simulink model "flythedrone"  (R2019b)
settings: Solver=FixedStepAuto  StartTime=0.0  StopTime=100  RelTol=1e-3
InitFcn:
  | load('BusDefinitions.mat')
values from neighbouring files (symbols this model uses):
  Kaileron = Kaileron(2:4)    [HW7_v2_matlab.m]
  Kelevator = Kelevator(2:4)    [HW7_v2_matlab.m]
  Krudder = Krudder(2)    [HW7_v2_matlab.m]
  Kthrust = lqr(Athrust, Bthrust, Qthrust, Rthrust)    [HW7_v2_matlab.m]
  M_motor = [1, 1, 1, -1;             1, 1, -1, 1;             1, -1, -1, -1;             1, -1, 1, 1 ]    [HW7_v2_matlab.m]
undefined symbols (not defined in the file or in its folder): A_s_double, A_s_single, B_s_double, B_s_single, C_double, C_single, codertarget, D_double, D_single, DiscIntNeverNeededParam, Discrete, omega_c, q_single, r_single, Time, Ts
libraries: ctrlSharedLib x5
settings Model: ExtModeTrigDuration=80  Creator=Sankalp Bhan  LastModifiedBy=cwhipp
settings OptimizationCC: PassReuseOutputArgsThreshold=0  MaxStackSize=64
settings DebuggingCC: ParameterTunabilityLossMsg=error  ArithmeticOperatorsInVariantConditions=warning
settings HardwareCC: ProdBitPerPointer=32  ProdBitPerSizeT=32  ProdBitPerPtrDiffT=32  ProdLargestAtomicInteger=Long  ProdWordSize=32  ProdHWDeviceType=ARM Compatible->ARM 9  UseEmbeddedCoderFeatures=off
settings SFSimCC: SimUseLocalCustomCode=off  MATLABDynamicMemAlloc=off
settings RTWCC: SystemTargetFile=ert.tlc  HardwareBoard=PARROT Mambo  TLCOptions="-aInlineSetEventsForThisBaseRateFcn=TLC_FALSE -aSuppressMultiTaskScheduler=TLC_FALSE   -aRateBasedStepFcn=1"  TemplateMakefile=ert_default_tmf  GenerateReport=on  RTWUseLocalCustomCode=off  Toolchain=Sourcery G++ Lite GNU Toolchain for Drones  LaunchReport=on
settings CodeAppCC: ForceParamTrailComments=on  OperatorAnnotations=on  StateflowObjectComments=on
settings ERTTargetCC: ERTCustomFileBanners=off  MatFileLogging=on  SupportContinuousTime=on  SupportNonInlinedSFcns=on  RemoveResetFunc=off  ModelStepFunctionPrototypeControlCompliant=off

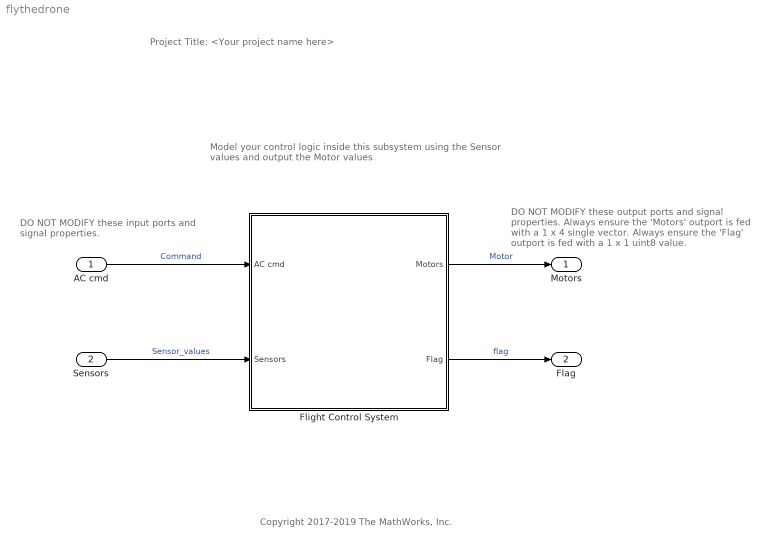
== system flythedrone ==
  note: Model your control logic inside this subsystem
      | using the Sensor values and output the
      | Motor values
  note: DO NOT MODIFY these output ports
      | and signal properties.
      |
      |
      |
      | Always ensure the 'Motors' outport
      | is fed with a 1 x 4 single vector.
      |
      |
      |
      |
      |
      | Always ensure the 'Flag' outport is
      | fed with a 1 x 1 uint8 value.
  note: DO NOT MODIFY these input
      | ports and signal properties.
  note: Copyright 2017-2019 The MathWorks, Inc.
  note: Project Title: <Your project name here>
  AC cmd : Inport  OutDataTypeStr=Bus: CommandBus  BusOutputAsStruct=on
  Sensors : Inport  Port=2  OutDataTypeStr=Bus: SensorsBus  BusOutputAsStruct=on
  Flight Control System : Subsystem  InitFcn=codertarget.parrot.internal.fcsSubsystemCallback(gcb);
  Motors : Outport  OutDataTypeStr=single  PortDimensions=[1 4]  VectorParamsAs1DForOutWhenUnconnected=off
  Flag : Outport  Port=2  OutDataTypeStr=uint8  PortDimensions=1  VectorParamsAs1DForOutWhenUnconnected=off
  wires:
  Flight Control System/1(Motors) -> Motors/1  "Motor"
  AC cmd/1 -> Flight Control System/1(AC cmd)  "Command"
  Sensors/1 -> Flight Control System/2(Sensors)  "Sensor_values"
  Flight Control System/2(Flag) -> Flag/1  "flag"

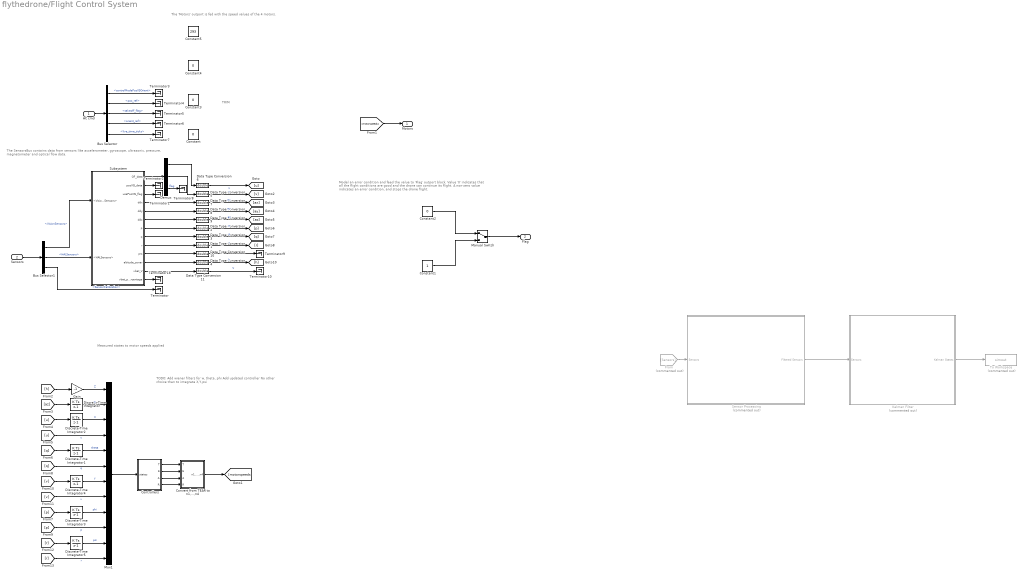
== system flythedrone/Flight Control System ==
  note: TODO:
      | Add wiener filters for w, theta, phi
      | Add updated controller
      |
      | No other choice than to integrate X,Y,psi
  note: Measured states to motor speeds applied
  note: TRIM
  note: The 'Motors' outport is fed with the speed values of the 4 motors.
  note: Model an error condition and feed the value to 'Flag' outport block.
      | Value '0' indicates that all the flight conditions are good and the drone
      | can continue its flight.
      | A non-zero value indicates an error condition, and stops the drone
      | flight.
  note: The SensorsBus contains data from sensors like
      | accelerometer, gyroscope, ultrasonic, pressure,
      | magnetometer and optical flow data.
  AC cmd : Inport
  Sensors : Inport  Port=2
  Bus Selector : BusSelector  OutputSignals=controlModePosVSOrient,pos_ref,takeoff_flag,orient_ref,live_time_ticks
  Bus Selector1 : BusSelector  OutputSignals=VisionSensors,HALSensors,SensorCalibration
  Constant : Constant  Value=0  SampleTime=Ts
  Constant1 : Constant  OutDataTypeStr=uint8
  Constant2 : Constant  Value=0  OutDataTypeStr=uint8
  Constant3 : Constant  Value=0  SampleTime=Ts
  Constant4 : Constant  Value=0  SampleTime=Ts
  Constant5 : Constant  Value=293  SampleTime=Ts
  Controllers : Subsystem
  Convert from TEAR to n1,...,n4 : Subsystem
  Data Type Conversion{1..11} (11 alike) : DataTypeConversion  OutDataTypeStr=double
  Demux : Demux  Outputs=3
  Discrete-Time Integrator{,1..5} (6 alike) : DiscreteIntegrator  SampleTime=-1  ICPrevOutput=DiscIntNeverNeededParam  ICPrevScaledInput=DiscIntNeverNeededParam
  From : From  Commented=on  GotoTag=Sensors
  Gain : Gain  Gain=-1
  Kalman Filter : Subsystem  Commented=on
  Manual Switch : ManualSwitch
  Mux1 : Mux  Inputs=12
  "Sensor Processing " : Subsystem  Commented=on
  Subsystem : Subsystem
  Terminator{,1..10,18} (12 alike) : Terminator
  To Workspace : ToWorkspace  Commented=on  VariableName=simout  SaveFormat=Structure With Time  SampleTime=-1
  Motors : Outport  VectorParamsAs1DForOutWhenUnconnected=off
  Flag : Outport  Port=2  VectorParamsAs1DForOutWhenUnconnected=off
  wires:
  AC cmd/1 -> Bus Selector/1
  Sensors/1 -> Bus Selector1/1
  Bus Selector/1 -> Terminator3/1  "<controlModePosVSOrient>"
  Bus Selector/2 -> Terminator4/1  "<pos_ref>"
  Bus Selector/3 -> Terminator5/1  "<takeoff_flag>"
  Bus Selector/4 -> Terminator6/1  "<orient_ref>"
  Bus Selector/5 -> Terminator7/1  "<live_time_ticks>"
  Manual Switch/1 -> Flag/1
  Constant2/1 -> Manual Switch/1
  Constant1/1 -> Manual Switch/2
  [motorspeeds] -> Motors/1
  Bus Selector1/1 -> Subsystem/1(<VisionSensors>)  "<VisionSensors>"
  Bus Selector1/2 -> Subsystem/2(<HALSensors>)  "<HALSensors>"
  Bus Selector1/3 -> Terminator/1  "<SensorCalibration>"
  Subsystem/1(OF_data) -> Demux/1
  Subsystem/4(ddx) -> Data Type Conversion7/1
  Subsystem/5(ddy) -> Data Type Conversion8/1
  Subsystem/6(ddz) -> Data Type Conversion9/1
  Subsystem/7(p) -> Data Type Conversion2/1
  Subsystem/9(r) -> Data Type Conversion1/1
  Subsystem/11(altitude_sonar) -> Data Type Conversion4/1
  Subsystem/12(vbat_V) -> Data Type Conversion11/1
  Subsystem/13(vbat_percentage) -> Terminator18/1
  Subsystem/8(q) -> Data Type Conversion3/1
  Subsystem/3(usePosVIS_flag) -> Terminator1/1
  Subsystem/2(posVIS_data) -> Terminator2/1
  Demux/1 -> Data Type Conversion6/1
  Demux/2 -> Data Type Conversion5/1
  Demux/3 -> Terminator8/1  "flag"
  Subsystem/10(prs) -> Data Type Conversion10/1
  Data Type Conversion1/1 -> [r]  "r"
  Data Type Conversion2/1 -> [p]  "p"
  Data Type Conversion3/1 -> [q]  "q"
  Data Type Conversion4/1 -> [h]  "h"
  Data Type Conversion5/1 -> [v]  "v"
  Data Type Conversion6/1 -> [u]  "u"
  Data Type Conversion7/1 -> [ax]  "ax"
  Data Type Conversion8/1 -> [ay]  "ay"
  Data Type Conversion9/1 -> [az]  "az"
  Data Type Conversion10/1 -> Terminator9/1
  Data Type Conversion11/1 -> Terminator10/1  "V"
  From/1 -> "Sensor Processing "/1(Sensors)
  "Sensor Processing "/1(Filtered Sensors) -> Kalman Filter/1(Sensors)
  Kalman Filter/1(Kalman States) -> To Workspace/1
  Mux1/1 -> Controllers/1(states)
  Controllers/3(A) -> Convert from TEAR to n1,...,n4/3(A)
  Controllers/4(R) -> Convert from TEAR to n1,...,n4/4(R)
  Controllers/1(T) -> Convert from TEAR to n1,...,n4/1(T)
  Controllers/2(E) -> Convert from TEAR to n1,...,n4/2(E)
  Convert from TEAR to n1,...,n4/1(n1,...,n4) -> [motorspeeds]
  [h] -> Gain/1
  Gain/1 -> Mux1/1  "Z"
  [az] -> Discrete-Time Integrator/1
  Discrete-Time Integrator/1 -> Mux1/2  "w"
  [u] -> Mux1/4  "u"
  Discrete-Time Integrator2/1 -> Mux1/3  "X"
  [u] -> Discrete-Time Integrator2/1
  [q] -> Discrete-Time Integrator1/1
  Discrete-Time Integrator1/1 -> Mux1/5  "theta"
  [q] -> Mux1/6  "q"
  Discrete-Time Integrator4/1 -> Mux1/7  "Y"
  [p] -> Mux1/10  "p"
  [p] -> Discrete-Time Integrator3/1
  Discrete-Time Integrator3/1 -> Mux1/9  "phi"
  [v] -> Discrete-Time Integrator4/1
  [v] -> Mux1/8  "v"
  [r] -> Discrete-Time Integrator5/1
  Discrete-Time Integrator5/1 -> Mux1/11  "psi"
  [r] -> Mux1/12  "r"

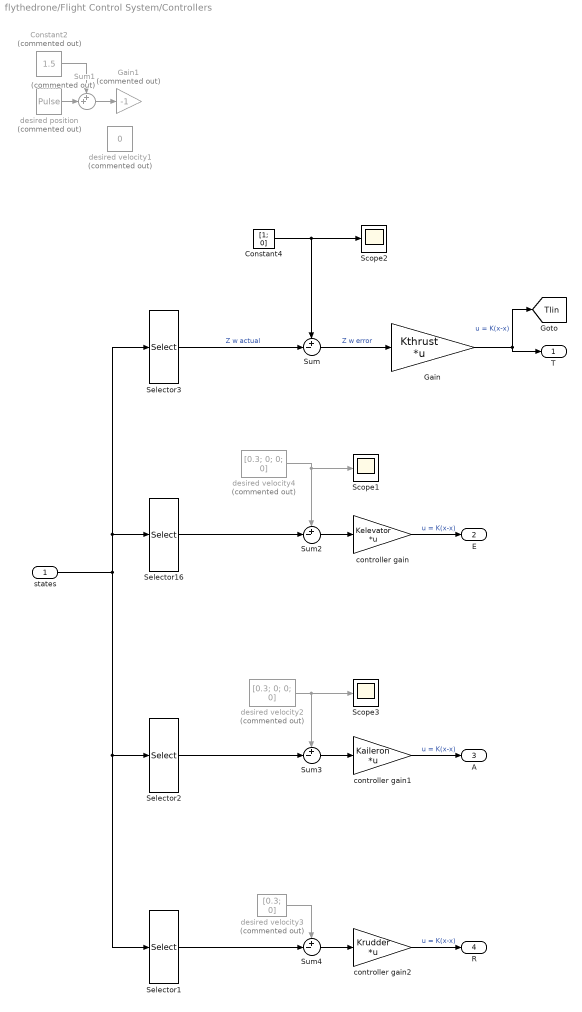
== system flythedrone/Flight Control System/Controllers ==
  states : Inport
  Constant2 : Constant  Commented=on  Value=1.5  SampleTime=0.05
  Constant4 : Constant  Value=[1; 0]  SampleTime=0.05
  Gain : Gain  Gain=Kthrust  Multiplication=Matrix(K*u)
  Gain1 : Gain  Commented=on  Gain=-1
  Scope1 : Scope
  Scope2 : Scope
  Scope3 : Scope
  Selector1 : Selector  InputPortWidth=12  IndexOptions=Index vector (dialog)  Indices=[11 12]  OutputSizes=1
  Selector16 : Selector  InputPortWidth=12  IndexOptions=Index vector (dialog)  Indices=[3 4 5 6]  OutputSizes=1
  Selector2 : Selector  InputPortWidth=12  IndexOptions=Index vector (dialog)  Indices=[7 8 9 10]  OutputSizes=1
  Selector3 : Selector  InputPortWidth=12  IndexOptions=Index vector (dialog)  Indices=[1 2]  OutputSizes=1
  Sum{,2..4} (4 alike) : Sum  Inputs=+-|
  Sum1 : Sum  Commented=on  Inputs=++|
  controller gain : Gain  Gain=Kelevator  Multiplication=Matrix(K*u)
  controller gain1 : Gain  Gain=Kaileron  Multiplication=Matrix(K*u)
  controller gain2 : Gain  Gain=Krudder  Multiplication=Matrix(K*u)
  desired position : DiscretePulseGenerator  Commented=on  PulseType=Time based  Amplitude=-1.5  Period=10  PulseWidth=50
  desired velocity1 : Constant  Commented=on  Value=0  SampleTime=0.05
  desired velocity2 : Constant  Commented=on  Value=[0.3; 0; 0; 0]  SampleTime=0.05
  desired velocity3 : Constant  Commented=on  Value=[0.3; 0]  SampleTime=0.05
  desired velocity4 : Constant  Commented=on  Value=[0.3; 0; 0; 0]  SampleTime=0.05
  T : Outport
  E : Outport  Port=2
  A : Outport  Port=3
  R : Outport  Port=4
  tag scope: Tlin=global
  wires:
  states/1 -> Selector16/1, Selector3/1, Selector2/1, Selector1/1
  Constant4/1 -> Scope2/1, Sum/1
  Sum/1 -> Gain/1  "Z w error"
  Gain/1 -> T/1, [Tlin]  "u = K(x-x)"
  desired velocity4/1 -> Scope1/1, Sum2/1
  Sum2/1 -> controller gain/1
  controller gain/1 -> E/1  "u = K(x-x)"
  controller gain1/1 -> A/1  "u = K(x-x)"
  Sum3/1 -> controller gain1/1
  controller gain2/1 -> R/1  "u = K(x-x)"
  Sum4/1 -> controller gain2/1
  desired velocity3/1 -> Sum4/1
  Selector3/1 -> Sum/2  "Z w actual"
  Selector16/1 -> Sum2/2
  Selector2/1 -> Sum3/2
  Selector1/1 -> Sum4/2
  Constant2/1 -> Sum1/1
  desired position/1 -> Sum1/2
  Sum1/1 -> Gain1/1
  desired velocity2/1 -> Sum3/1, Scope3/1

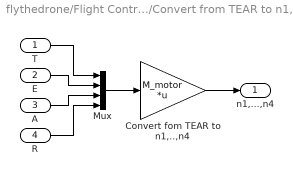
== system flythedrone/Flight Control System/Convert from TEAR to n1,...,n4 ==
  T : Inport
  E : Inport  Port=2
  A : Inport  Port=3
  R : Inport  Port=4
  Convert fom TEAR to n1,..,n4 : Gain  Gain=M_motor  Multiplication=Matrix(K*u)
  Mux : Mux
  n1,...,n4 : Outport
  wires:
  Convert fom TEAR to n1,..,n4/1 -> n1,...,n4/1
  Mux/1 -> Convert fom TEAR to n1,..,n4/1
  T/1 -> Mux/1
  E/1 -> Mux/2
  A/1 -> Mux/3
  R/1 -> Mux/4

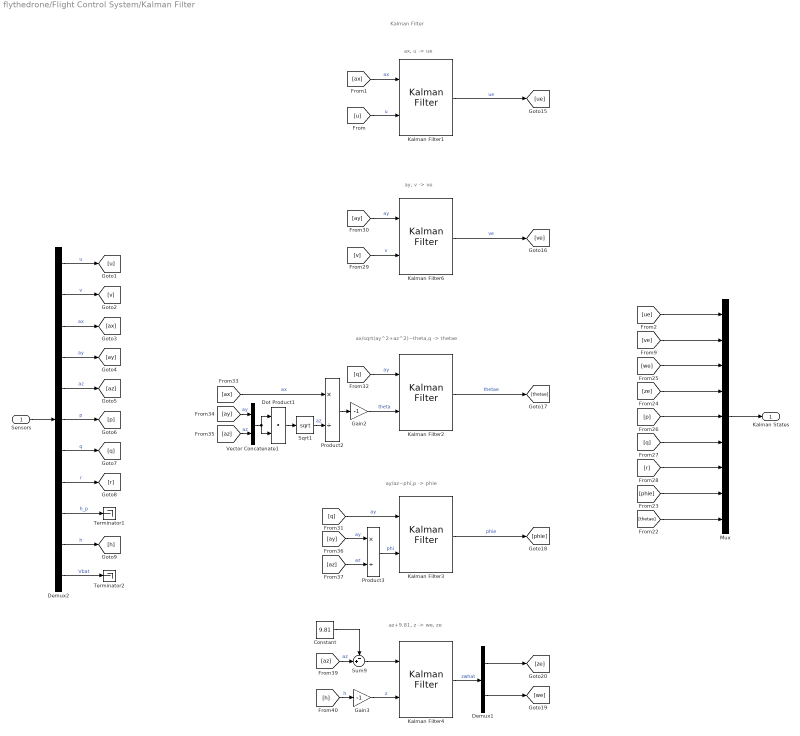
== system flythedrone/Flight Control System/Kalman Filter ==
  note: ay/az~phi,p -> phie
  note: ax/sqrt(ay^2+az^2)~theta,q -> thetae
  note: ax, u -> ue
  note: az+9.81, z -> we, ze
  note: ay, v -> ve
  note: Kalman Filter
  Sensors : Inport
  Constant : Constant  Value=9.81  SampleTime=0.005
  Demux1 : Demux  Outputs=2
  Demux2 : Demux  Outputs=11
  Dot Product1 : DotProduct  OutMin=0.0001  InputSameDT=on  OutDataTypeStr=Inherit: Inherit via internal rule
  Gain2 : Gain  Gain=-1
  Gain3 : Gain  Gain=-1
  Kalman Filter{1..3,6} (4 alike) : ctrlSharedLib/Kalman Filter  TimeDomain=Discrete-Time  UseCurrentEstimator=on  ModelSource=Individual A, B, C, D matrices  ModelSourceVariable=ss(0.95,1,1,0,1)  A=A_s_single  B=B_s_single  C=C_single  D=D_single  NumberOfStates=1  NumberOfInputs=1  NumberOfOutputs=1  InitialEstimateSource=Dialog  X0=[0]  P0=10  UseK=off  UseGH=off  NumberOfProcessNoiseInputs=1  G=1  TimeInvariantG=on  H=0  TimeInvariantH=on  Q=[1]*q_single  TimeInvariantQ=on  R=[1]*r_single*10000  TimeInvariantR=on  N=0  TimeInvariantN=on  AddInputPort=on  AddEnablePort=off  OutputEstimatedY=off  OutputP=off  Ts=Ts
      settings: SourceProductBaseCode=CT
  Kalman Filter4 : ctrlSharedLib/Kalman Filter  TimeDomain=Discrete-Time  UseCurrentEstimator=on  ModelSource=Individual A, B, C, D matrices  ModelSourceVariable=ss(0.95,1,1,0,1)  A=A_s_double  B=B_s_double  C=C_double  D=D_double  NumberOfStates=1  NumberOfInputs=1  NumberOfOutputs=1  InitialEstimateSource=Dialog  X0=[0]  P0=10  UseK=off  UseGH=off  NumberOfProcessNoiseInputs=1  G=1  TimeInvariantG=on  H=0  TimeInvariantH=on  Q=[0 0; 0 1]*q_single  TimeInvariantQ=on  R=[1]*r_single*10000  TimeInvariantR=on  N=0  TimeInvariantN=on  AddInputPort=on  AddEnablePort=off  OutputEstimatedY=off  OutputP=off  Ts=Ts
      settings: SourceProductBaseCode=CT
  Mux : Mux  Inputs=9
  Product2 : Product  Inputs=*/
  Product3 : Product  Inputs=*/
  Sqrt1 : Sqrt  SaturateOnIntegerOverflow=on
  Sum9 : Sum  Inputs=-+|
  Terminator1 : Terminator
  Terminator2 : Terminator
  Vector Concatenate1 : Concatenate
  Kalman States : Outport
  wires:
  Demux2/9 -> Terminator1/1  "h_p"
  Demux2/1 -> [u]  "u"
  Demux2/4 -> [ay]  "ay"
  Demux2/3 -> [ax]  "ax"
  Sensors/1 -> Demux2/1
  Demux2/2 -> [v]  "v"
  Demux2/10 -> [h]  "h"
  Demux2/5 -> [az]  "az"
  Demux2/7 -> [q]  "q"
  Demux2/8 -> [r]  "r"
  Demux2/6 -> [p]  "p"
  Demux2/11 -> Terminator2/1  "Vbat"
  [ue] -> Mux/1
  [ve] -> Mux/2
  [we] -> Mux/3
  [ze] -> Mux/4
  Mux/1 -> Kalman States/1
  [r] -> Mux/7
  [q] -> Mux/6
  [p] -> Mux/5
  [phie] -> Mux/8
  [thetae] -> Mux/9
  Sqrt1/1 -> Product2/2  "az"
  Gain3/1 -> Kalman Filter4/2  "z"
  Kalman Filter4/1 -> Demux1/1  "zwhat"
  [ax] -> Product2/1  "ax"
  [v] -> Kalman Filter6/2  "v"
  Kalman Filter2/1 -> [thetae]  "thetae"
  [u] -> Kalman Filter1/2  "u"
  [ay] -> Kalman Filter6/1  "ay"
  Gain2/1 -> Kalman Filter2/2  "theta"
  [ay] -> Product3/1  "ay"
  Dot Product1/1 -> Sqrt1/1
  Product2/1 -> Gain2/1
  Demux1/2 -> [we]
  [ay] -> Vector Concatenate1/1  "ay"
  [az] -> Vector Concatenate1/2  "az"
  Vector Concatenate1/1 -> Dot Product1/1, Dot Product1/2
  Product3/1 -> Kalman Filter3/2  "phi"
  Demux1/1 -> [ze]
  Kalman Filter6/1 -> [ve]  "ve"
  [h] -> Gain3/1  "h"
  [q] -> Kalman Filter3/1  "ay"
  Kalman Filter1/1 -> [ue]  "ue"
  [q] -> Kalman Filter2/1  "ay"
  Kalman Filter3/1 -> [phie]  "phie"
  [az] -> Product3/2  "az"
  Sum9/1 -> Kalman Filter4/1
  Constant/1 -> Sum9/1
  [az] -> Sum9/2  "az"
  [ax] -> Kalman Filter1/1  "ax"

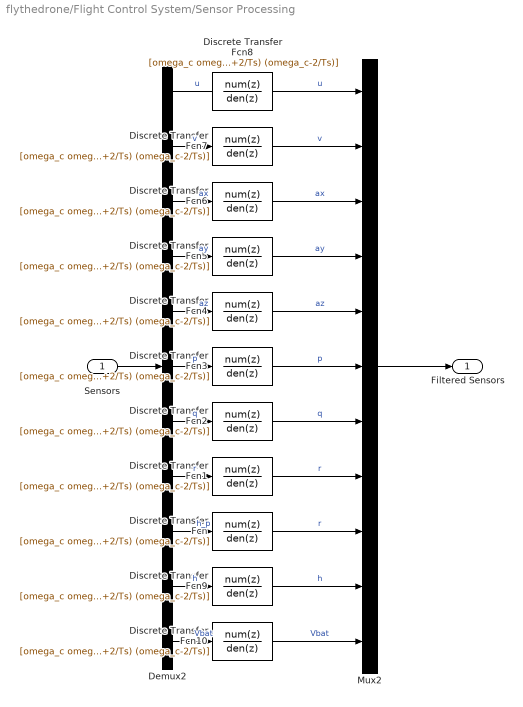
== system flythedrone/Flight Control System/Sensor Processing  ==
  Sensors : Inport
  Demux2 : Demux  Outputs=11
  Discrete Transfer Fcn{,1..10} (11 alike) : DiscreteTransferFcn  Numerator=[omega_c omega_c]  Denominator=[(omega_c+2/Ts) (omega_c-2/Ts)]  SampleTime=0.005
  Mux2 : Mux  Inputs=11
  Filtered Sensors : Outport
  wires:
  Mux2/1 -> Filtered Sensors/1
  Demux2/2 -> Discrete Transfer Fcn7/1  "v"
  Discrete Transfer Fcn9/1 -> Mux2/10  "h"
  Demux2/11 -> Discrete Transfer Fcn10/1  "Vbat"
  Sensors/1 -> Demux2/1
  Demux2/6 -> Discrete Transfer Fcn3/1  "p"
  Discrete Transfer Fcn2/1 -> Mux2/7  "q"
  Demux2/3 -> Discrete Transfer Fcn6/1  "ax"
  Demux2/4 -> Discrete Transfer Fcn5/1  "ay"
  Demux2/1 -> ?  "u"
  Discrete Transfer Fcn7/1 -> Mux2/2  "v"
  Demux2/8 -> Discrete Transfer Fcn1/1  "r"
  Discrete Transfer Fcn8/1 -> Mux2/1  "u"
  Discrete Transfer Fcn5/1 -> Mux2/4  "ay"
  Discrete Transfer Fcn1/1 -> Mux2/8  "r"
  Demux2/10 -> Discrete Transfer Fcn9/1  "h"
  Discrete Transfer Fcn4/1 -> Mux2/5  "az"
  Demux2/7 -> Discrete Transfer Fcn2/1  "q"
  Discrete Transfer Fcn10/1 -> Mux2/11  "Vbat"
  Discrete Transfer Fcn3/1 -> Mux2/6  "p"
  Demux2/5 -> Discrete Transfer Fcn4/1  "az"
  Discrete Transfer Fcn6/1 -> Mux2/3  "ax"
  Demux2/9 -> Discrete Transfer Fcn/1  "h_p"
  Discrete Transfer Fcn/1 -> Mux2/9  "r"

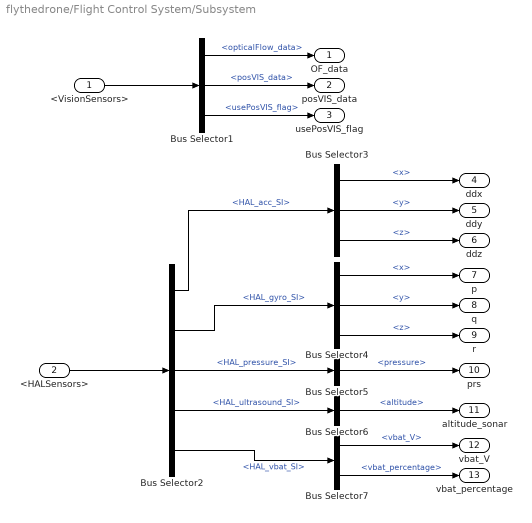
== system flythedrone/Flight Control System/Subsystem ==
  <VisionSensors> : Inport
  <HALSensors> : Inport  Port=2
  Bus Selector1 : BusSelector  OutputSignals=opticalFlow_data,posVIS_data,usePosVIS_flag
  Bus Selector2 : BusSelector  OutputSignals=HAL_acc_SI,HAL_gyro_SI,HAL_pressure_SI,HAL_ultrasound_SI,HAL_vbat_SI
  Bus Selector3 : BusSelector  OutputSignals=x,y,z
  Bus Selector4 : BusSelector  OutputSignals=x,y,z
  Bus Selector5 : BusSelector  OutputSignals=pressure
  Bus Selector6 : BusSelector  OutputSignals=altitude
  Bus Selector7 : BusSelector  OutputSignals=vbat_V,vbat_percentage
  OF_data : Outport  VectorParamsAs1DForOutWhenUnconnected=off
  posVIS_data : Outport  Port=2  VectorParamsAs1DForOutWhenUnconnected=off
  usePosVIS_flag : Outport  Port=3  VectorParamsAs1DForOutWhenUnconnected=off
  ddx : Outport  Port=4  VectorParamsAs1DForOutWhenUnconnected=off
  ddy : Outport  Port=5  VectorParamsAs1DForOutWhenUnconnected=off
  ddz : Outport  Port=6  VectorParamsAs1DForOutWhenUnconnected=off
  p : Outport  Port=7  VectorParamsAs1DForOutWhenUnconnected=off
  q : Outport  Port=8  VectorParamsAs1DForOutWhenUnconnected=off
  r : Outport  Port=9  VectorParamsAs1DForOutWhenUnconnected=off
  prs : Outport  Port=10  VectorParamsAs1DForOutWhenUnconnected=off
  altitude_sonar : Outport  Port=11  VectorParamsAs1DForOutWhenUnconnected=off
  vbat_V : Outport  Port=12  VectorParamsAs1DForOutWhenUnconnected=off
  vbat_percentage : Outport  Port=13  VectorParamsAs1DForOutWhenUnconnected=off
  wires:
  <VisionSensors>/1 -> Bus Selector1/1
  <HALSensors>/1 -> Bus Selector2/1
  Bus Selector1/1 -> OF_data/1  "<opticalFlow_data>"
  Bus Selector1/2 -> posVIS_data/1  "<posVIS_data>"
  Bus Selector1/3 -> usePosVIS_flag/1  "<usePosVIS_flag>"
  Bus Selector2/1 -> Bus Selector3/1  "<HAL_acc_SI>"
  Bus Selector2/2 -> Bus Selector4/1  "<HAL_gyro_SI>"
  Bus Selector2/3 -> Bus Selector5/1  "<HAL_pressure_SI>"
  Bus Selector2/4 -> Bus Selector6/1  "<HAL_ultrasound_SI>"
  Bus Selector2/5 -> Bus Selector7/1  "<HAL_vbat_SI>"
  Bus Selector3/1 -> ddx/1  "<x>"
  Bus Selector3/2 -> ddy/1  "<y>"
  Bus Selector3/3 -> ddz/1  "<z>"
  Bus Selector4/2 -> q/1  "<y>"
  Bus Selector4/1 -> p/1  "<x>"
  Bus Selector4/3 -> r/1  "<z>"
  Bus Selector5/1 -> prs/1  "<pressure>"
  Bus Selector6/1 -> altitude_sonar/1  "<altitude>"
  Bus Selector7/1 -> vbat_V/1  "<vbat_V>"
  Bus Selector7/2 -> vbat_percentage/1  "<vbat_percentage>"
